simulink model "gm_rampa_ref"  (R2017a)
settings: Solver=FixedStepDiscrete  StartTime=0.0  StopTime=10.0  FixedStep=0.001  MaxStep=1e-4  RelTol=1e-3
undefined symbols (not defined in the file or in its folder): N
libraries: simulink x1
settings Model: Creator=Windows  LastModifiedBy=Windows
settings DataIOCC: LimitDataPoints=on  SaveOutput=off  SaveTime=off
settings OptimizationCC: BlockReduction=off  ConditionallyExecuteInputs=off  DefaultParameterBehavior=Inlined
settings DebuggingCC: AlgebraicLoopMsg=error  InheritedTsInSrcMsg=none  SingleTaskRateTransMsg=error  AllowSymbolicDim=off  StrictBusMsg=ErrorOnBusTreatedAsVector  SFUnexpectedBacktrackingDiag=warning  SFNoUnconditionalDefaultTransitionDiag=warning  SFExecutionAtInitializationDiag=none
settings HardwareCC: ProdLargestAtomicFloat=None  ProdLongLongMode=on  ProdHWDeviceType=Generic->Custom  TargetBitPerPointer=64  TargetBitPerSizeT=64  TargetBitPerPtrDiffT=64  TargetLongLongMode=on  TargetIntDivRoundTo=Zero  TargetEndianess=LittleEndian  TargetWordSize=64  TargetHWDeviceType=Generic->Custom
settings RTWCC: SystemTargetFile=systemverilog_dpi_grt.tlc  TemplateMakefile=systemverilog_dpi_grt_default_tmf  Description=SystemVerilog DPI Component Generator  RTWVerbose=off  BuildConfiguration=Faster Runs
settings CodeAppCC: MaxIdLength=256
settings DPIGRTTargetCC: TargetFcnLib=ansi_tfl_table_tmw.mat  GenFloatMathFcnCalls=NOT IN USE  TargetLangStandard=C89/C90 (ANSI)  CodeReplacementLibrary=None  UtilityFuncGeneration=Auto  MultiwordTypeDef=System defined  MultiwordLength=2048  GenerateFullHeader=on  InferredTypesCompatibility=off  GenerateSampleERTMain=off  GenerateTestInterfaces=off  ModelReferenceCompliant=on  ParMdlRefBuildCompliant=on  CompOptLevelCompliant=off  ConcurrentExecutionCompliant=off  IncludeMdlTerminateFcn=on  GeneratePreprocessorConditionals=Use local settings  CombineOutputUpdateFcns=off  CombineSignalStateStructs=on  SuppressErrorStatus=off  ERTFirstTimeCompliant=off  IncludeFileDelimiter=Auto  ERTCustomFileBanners=off  SupportAbsoluteTime=on  LogVarNameModifier=rt_  MatFileLogging=off  MultiInstanceERTCode=on  CodeInterfacePackaging=Reusable function  SupportNonFinite=on  SupportComplex=on  PurelyIntegerCode=off  SupportContinuousTime=on  SupportNonInlinedSFcns=on  RemoveDisableFunc=off  RemoveResetFunc=off  SupportVariableSizeSignals=off  ParenthesesLevel=Nominal  CastingMode=Nominal  MATLABClassNameForMDSCustomization=Simulink.SoftwareTarget.TargetSpecificTriggerConfigurationBase  ModelStepFunctionPrototypeControlCompliant=off  CPPClassGenCompliant=off  AutosarCompliant=off  MDXCompliant=off  GRTInterface=off  GenerateAllocFcn=on  UseToolchainInfoCompliant=on  GenerateSharedConstants=on  CoderGroups=[]  AccessMethods=[]  LookupTableObjectStructAxisOrder=1,2,3,4,...  RTWCAPISignals=on  RTWCAPIParams=off  RTWCAPIStates=off  RTWCAPIRootIO=off  ExtMode=off  ExtModeTransport=0  ExtModeStaticAlloc=off  ExtModeStaticAllocSize=1000000  ExtModeTesting=off  ExtModeMexFile=ext_comm  GenerateASAP2=off  MultiInstanceErrorCode=Error  DPICustomizeSystemVerilogCode=on  DPISystemVerilogTemplate=hdlverifier_dpitb_template.vgt  DPIGenerateTestBench=off  DPITestPointAccessFcnInterface=None
settings ConfigComp: CovScope=ReferencedModels  CovMetricSettings=dw  CovHtmlReporting=on  CovSaveCumulativeToWorkspaceVar=on  CovSaveSingleToWorkspaceVar=on  CovExternalEMLEnable=off  CovSFcnEnable=off

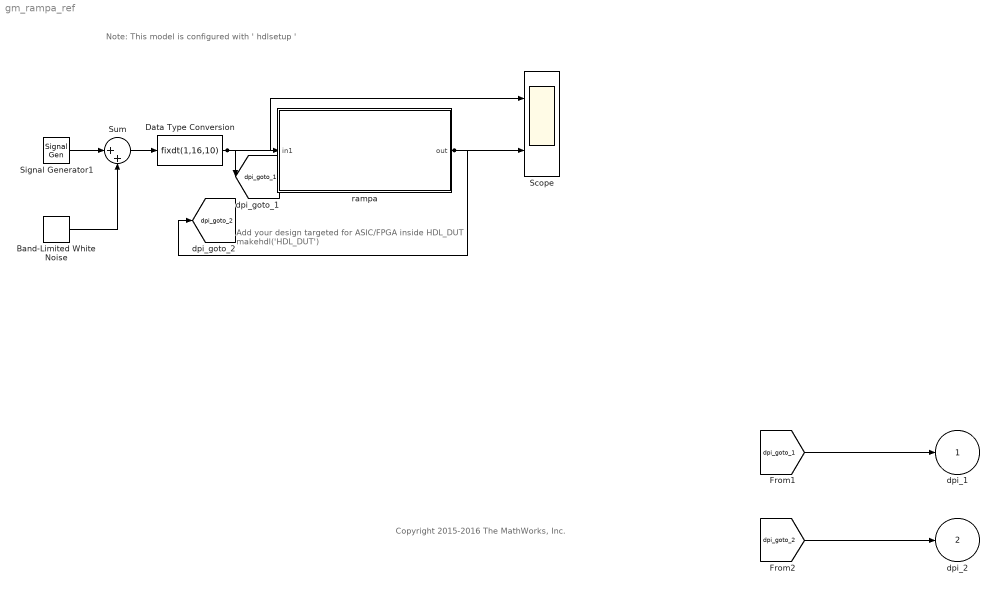
== system gm_rampa_ref ==
  note: Note: This model is configured with ' hdlsetup '
  note: Add your design targeted for ASIC/FPGA inside HDL_DUT
      | makehdl('HDL_DUT')
  note: Copyright 2015-2016 The MathWorks, Inc.
  Band-Limited White Noise : simulink/Sources/Band-Limited White Noise  Cov=[0.001]  Ts=0.001  seed=[23341]
  Data Type Conversion : DataTypeConversion  OutDataTypeStr=fixdt(1,16,10)
  Scope : Scope  NumInputPorts=2
  Signal Generator1 : SignalGenerator  Frequency=2000
  Sum : Sum  Inputs=|++
  rampa : Subsystem
  dpi_1 : Outport
  dpi_2 : Outport  Port=2  OutDataTypeStr=fixdt(1,16,10)
  tag scope: dpi_goto_1=global, dpi_goto_2=global
  wires:
  Data Type Conversion/1 -> Scope/1, rampa/1(in1), [dpi_goto_1]
  Signal Generator1/1 -> Sum/1
  Sum/1 -> Data Type Conversion/1
  Band-Limited White Noise/1 -> Sum/2
  rampa/1(out) -> Scope/2, [dpi_goto_2]
  [dpi_goto_1] -> dpi_1/1
  [dpi_goto_2] -> dpi_2/1

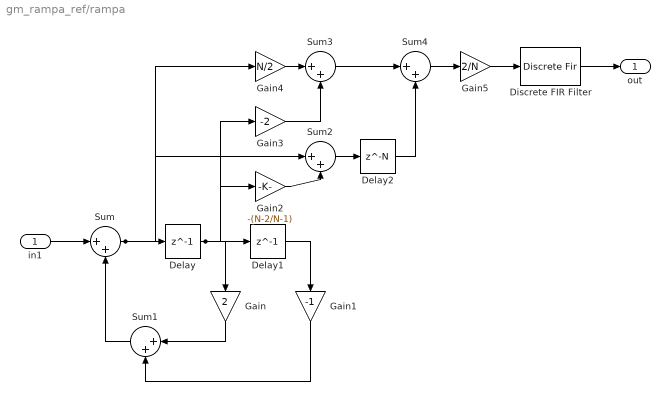
== system gm_rampa_ref/rampa ==
  in1 : Inport  OutDataTypeStr=fixdt(1, 16, 10)  SampleTime=0
  Delay : Delay  DelayLength=1
  Delay1 : Delay  DelayLength=1
  Delay2 : Delay  DelayLength=N
  Discrete FIR Filter : DiscreteFir  Coefficients=[0.1095 0.1047 0.1000 0.0952 0.0904 0.0857 0.0809 0.0761 0.0714 0.0666 0.0619 0.0571 0.0523 0.0476 0.0428 0.0380 0.0333 0.0285 0.0238 0.0190 0.0142 0.0095 0.0047 0 -0.0047 -0.0095 -0.0142 -0.0190 -0.0238 -0.0285 -0.0333 -0.0380 -0.0428 -0.0476 -0.0523]  CoefDataTypeStr=fixdt(1,16,10)  ProductDataTypeStr=fixdt(1,16,10)  AccumDataTypeStr=fixdt(1,16,10)  OutDataTypeStr=fixdt(1,16,10)
  Gain : Gain  Gain=2
  Gain1 : Gain  Gain=-1
  Gain2 : Gain  Gain=-(N-2/N-1)
  Gain3 : Gain  Gain=-2
  Gain4 : Gain  Gain=N/2
  Gain5 : Gain  Gain=2/N
  Sum{,1..4} (5 alike) : Sum  Inputs=|++  AccumDataTypeStr=fixdt(1,16,10)  OutDataTypeStr=fixdt(1,16,10)
  out : Outport  OutDataTypeStr=fixdt(1,16,10)
  wires:
  Sum4/1 -> Gain5/1
  Sum3/1 -> Sum4/1
  Sum2/1 -> Delay2/1
  Sum1/1 -> Sum/2
  Sum/1 -> Delay/1, Gain4/1, Sum2/1
  Gain5/1 -> Discrete FIR Filter/1
  Gain4/1 -> Sum3/1
  Gain3/1 -> Sum3/2
  Gain2/1 -> Sum2/2
  Gain1/1 -> Sum1/2
  Gain/1 -> Sum1/1
  Discrete FIR Filter/1 -> out/1
  Delay2/1 -> Sum4/2
  Delay1/1 -> Gain1/1
  Delay/1 -> Delay1/1, Gain/1, Gain2/1, Gain3/1
  in1/1 -> Sum/1
